simulink library "constantBasisParameters_varGeom_cl"  (R2020a)
settings: Solver=VariableStepAuto  StartTime=0.0  StopTime=10.0  RelTol=1e-3
values from neighbouring files (symbols this model uses):
  HILVLCONTROLLER = 'constantBasisParameters_varGeom'    [varGeom.mat]    (also in varGeom_bs.m)
  hiLvlCtrl = CTR.controller    [varGeom_bs.m]
undefined symbols (not defined in the file or in its folder): initializeBussesFromBlock
settings Model: Creator=mcobb  LastModifiedBy=andre
settings DataIOCC: ReturnWorkspaceOutputs=off
settings DebuggingCC: ArithmeticOperatorsInVariantConditions=warning
settings SFSimCC: CustomCodeUndefinedFunction=UseInterfaceOnly

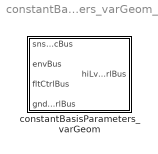
== system constantBasisParameters_varGeom_cl ==
  constantBasisParameters_varGeom : Subsystem  LoadFcn=initializeBussesFromBlock(gcb)  InitFcn=initializeBussesFromBlock(gcb)  StartFcn=initializeBussesFromBlock(gcb)  VariantControl=strcmpi(HILVLCONTROLLER,'constantBasisParameters')  mask{hiLvlCtrl=hiLvlCtrl}
      mask prompts: hiLvlCtrl "Hi-level controller"

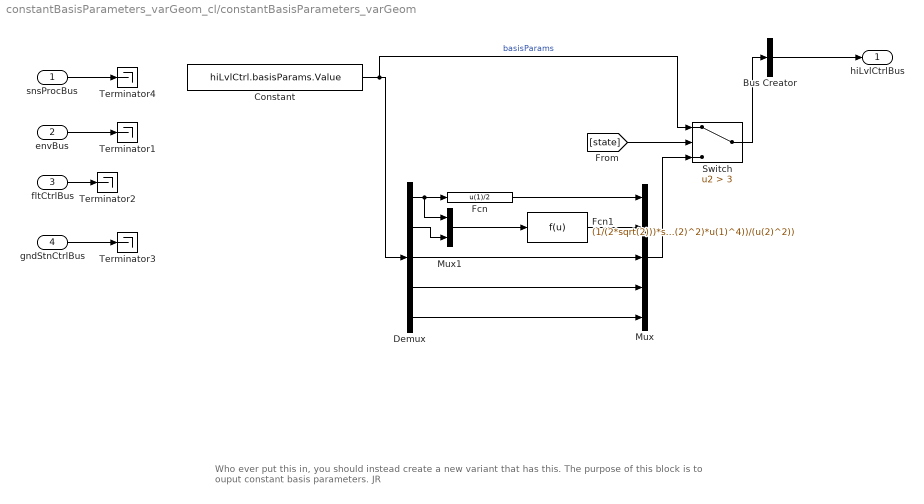
== system constantBasisParameters_varGeom_cl/constantBasisParameters_varGeom ==
  note: Who ever put this in, you should instead create a new variant that has this. The purpose of this block is to ouput constant basis parameters. JR
  snsProcBus : Inport  OutDataTypeStr=Bus: sensorsProcessingBus
  envBus : Inport  Port=2  OutDataTypeStr=Bus: envBus
  fltCtrlBus : Inport  Port=3  OutDataTypeStr=Bus: fltCtrlBus
  gndStnCtrlBus : Inport  Port=4  OutDataTypeStr=Bus: gndStnCtrlBus
  Bus Creator : BusCreator  Inputs=1  OutDataTypeStr=Bus: hiLvlCtrlBus
  Constant : Constant  Value=hiLvlCtrl.basisParams.Value
  Demux : Demux  Outputs=5
  Fcn : Fcn  Expr=u(1)/2
  Fcn1 : Fcn  Expr=(1/(2*sqrt(2)))*sqrt(-u(1)^2+sqrt((u(2)^2*(4+u(2)^2)*u(1)^4))/(u(2)^2))
  Mux : Mux  Inputs=5
  Mux1 : Mux  Inputs=2
  Switch : Switch  Criteria=u2 > Threshold  Threshold=3
  Terminator{1..4} (4 alike) : Terminator
  hiLvlCtrlBus : Outport  OutDataTypeStr=Bus: hiLvlCtrlBus  VectorParamsAs1DForOutWhenUnconnected=off
  wires:
  envBus/1 -> Terminator1/1
  gndStnCtrlBus/1 -> Terminator3/1
  Bus Creator/1 -> hiLvlCtrlBus/1
  fltCtrlBus/1 -> Terminator2/1
  Constant/1 -> Switch/1, Demux/1  "basisParams"
  snsProcBus/1 -> Terminator4/1
  Demux/5 -> Mux/5
  Demux/4 -> Mux/4
  Demux/3 -> Mux/3
  Demux/1 -> Mux1/1, Fcn/1
  Fcn/1 -> Mux/1
  Demux/2 -> Mux1/2
  Mux1/1 -> Fcn1/1
  Fcn1/1 -> Mux/2
  Mux/1 -> Switch/3
  Switch/1 -> Bus Creator/1
  [state] -> Switch/2
